simulink subsystem "ScaleParamToWavelen"  (R2024a)
settings: Solver=VariableStepAuto  StartTime=0.0  StopTime=10.0  RelTol=1e-3
undefined symbols (not defined in the file or in its folder): wave_len
settings Model: Creator=david  LastModifiedBy=dfurodet

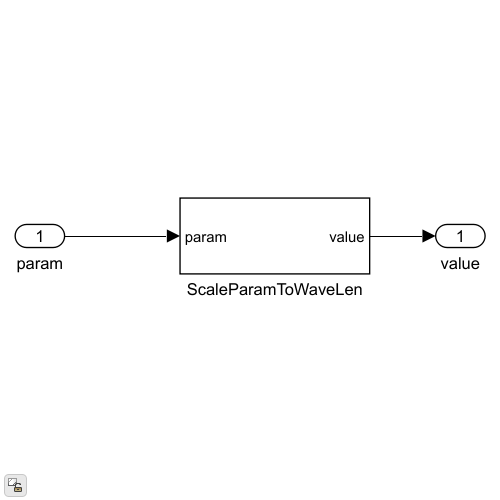
[thumbnail: Simulink's stored preview of the top-level diagram]
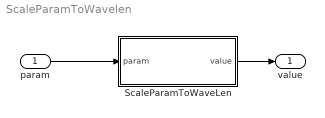
== system ScaleParamToWavelen ==
  param : Inport
  ScaleParamToWaveLen : Subsystem
  value : Outport
  wires:
  ScaleParamToWaveLen/1(value) -> value/1
  param/1 -> ScaleParamToWaveLen/1(param)

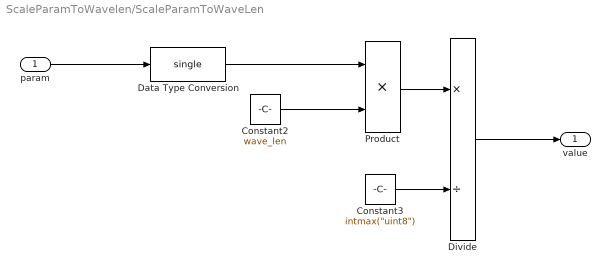
== system ScaleParamToWavelen/ScaleParamToWaveLen ==
  param : Inport
  Constant2 : Constant  Value=wave_len  OutDataTypeStr=single
  Constant3 : Constant  Value="intmax(\"uint8\")"
  Data Type Conversion : DataTypeConversion  OutDataTypeStr=single  SaturateOnIntegerOverflow=off  RndMeth=Floor
  Divide : Product  Inputs=*/
  Product : Product
  value : Outport
  wires:
  Data Type Conversion/1 -> Product/1
  Divide/1 -> value/1
  Product/1 -> Divide/1
  param/1 -> Data Type Conversion/1
  Constant3/1 -> Divide/2
  Constant2/1 -> Product/2
